simulink model "Gainbarcreator"  (R2017a)
settings: Solver=VariableStepAuto  StartTime=0.0  StopTime=10.0  RelTol=1e-3
settings Model: Creator=Administrator  LastModifiedBy=Administrator

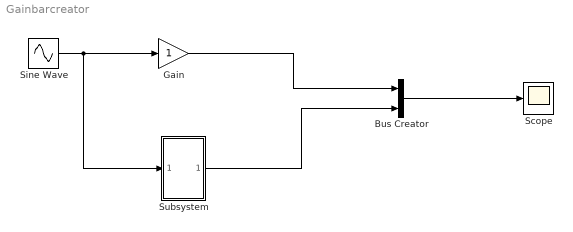
== system Gainbarcreator ==
  Bus Creator : BusCreator  Inputs=2
  Gain : Gain
  Scope : Scope
  Sine Wave : Sin  SampleTime=0
  Subsystem : Subsystem
  wires:
  Sine Wave/1 -> Subsystem/1(In1), Gain/1
  Gain/1 -> Bus Creator/1
  Subsystem/1(Out1) -> Bus Creator/2
  Bus Creator/1 -> Scope/1

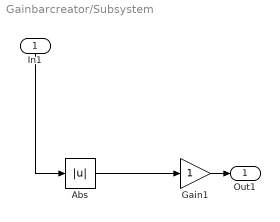
== system Gainbarcreator/Subsystem ==
  In1 : Inport
  Abs : Abs
  Gain1 : Gain
  Out1 : Outport
  wires:
  Abs/1 -> Gain1/1
  Gain1/1 -> Out1/1
  In1/1 -> Abs/1
